simulink model "fourdrive_test"  (R2022b)
settings: Solver=FixedStepDiscrete  StartTime=0.0  StopTime=10.0  FixedStep=0.001  RelTol=1e-3  EnableMultiTasking=on
PreLoadFcn:
  | PowerOn_data
InitFcn:
  | EcoCoder_PreCheckLic();
undefined symbols (not defined in the file or in its folder): HV_Botton, Inverter_Button, SC_Closed
libraries: CoderSF_BSW_Libs x113, SF_CanService_Libs x24, CoderSF_ADC2Volt_Libs x10, simulink x2
(part 2 of 2)

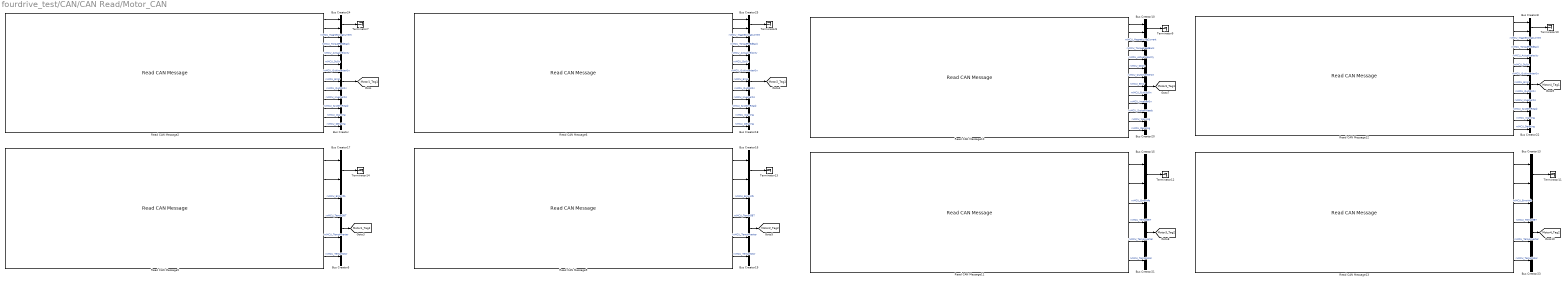
== system fourdrive_test/CAN/CAN Read/Motor_CAN ==
  Bus Creator{,18,20,22} (4 alike) : BusCreator  Inputs=11
  Bus Creator{8,10,13,15..17,24..25} (8 alike) : BusCreator  Inputs=2
  Bus Creator{5,19,21,23} (4 alike) : BusCreator  Inputs=4
  Read CAN Message10 : SF_CanService_Libs/Read CAN Message  typeCAN=Connected  channel=CAN_D  mEn=off  msgInfo=Motor_Can_All  msgItermStore=MCU_287_RL  msgIterm=MCU_287_RL  valid=on  stale=on  motoBit=off  setSignalName=on  flgCustomMonitorVariableRules=on  defineSignalName=off  prefixSignal='rx'  flgValTest=off  flgNoFixed=on  tSample=Task_Inherit  modeCode=Parameterless
  Read CAN Message11 : SF_CanService_Libs/Read CAN Message  typeCAN=Connected  channel=CAN_D  mEn=off  msgInfo=Motor_Can_All  msgItermStore=MCU_289_RL  msgIterm=MCU_289_RL  valid=on  stale=on  motoBit=off  setSignalName=on  flgCustomMonitorVariableRules=on  defineSignalName=off  prefixSignal='rx'  flgValTest=off  flgNoFixed=on  tSample=Task_Inherit  modeCode=Parameterless
  Read CAN Message12 : SF_CanService_Libs/Read CAN Message  typeCAN=Connected  channel=CAN_D  mEn=off  msgInfo=Motor_Can_All  msgItermStore=MCU_288_RR  msgIterm=MCU_288_RR  valid=on  stale=on  motoBit=off  setSignalName=on  flgCustomMonitorVariableRules=on  defineSignalName=off  prefixSignal='rx'  flgValTest=off  flgNoFixed=on  tSample=Task_Inherit  modeCode=Parameterless
  Read CAN Message13 : SF_CanService_Libs/Read CAN Message  typeCAN=Connected  channel=CAN_D  mEn=off  msgInfo=Motor_Can_All  msgItermStore=MCU_28A_RR  msgIterm=MCU_28A_RR  valid=on  stale=on  motoBit=off  setSignalName=on  flgCustomMonitorVariableRules=on  defineSignalName=off  prefixSignal='rx'  flgValTest=off  flgNoFixed=on  tSample=Task_Inherit  modeCode=Parameterless
  Read CAN Message2 : SF_CanService_Libs/Read CAN Message  typeCAN=Connected  channel=CAN_C  mEn=off  msgInfo=Motor_Can_All  msgItermStore=MCU_283_FL  msgIterm=MCU_283_FL  valid=on  stale=on  motoBit=off  setSignalName=on  flgCustomMonitorVariableRules=on  defineSignalName=off  prefixSignal='rx'  flgValTest=off  flgNoFixed=on  tSample=Task_Inherit  modeCode=Parameterless
  Read CAN Message5 : SF_CanService_Libs/Read CAN Message  typeCAN=Connected  channel=CAN_C  mEn=off  msgInfo=Motor_Can_All  msgItermStore=MCU_285_FL  msgIterm=MCU_285_FL  valid=on  stale=on  motoBit=off  setSignalName=on  flgCustomMonitorVariableRules=on  defineSignalName=off  prefixSignal='rx'  flgValTest=off  flgNoFixed=on  tSample=Task_Inherit  modeCode=Parameterless
  Read CAN Message6 : SF_CanService_Libs/Read CAN Message  typeCAN=Connected  channel=CAN_C  mEn=off  msgInfo=Motor_Can_All  msgItermStore=MCU_284_FR  msgIterm=MCU_284_FR  valid=on  stale=on  motoBit=off  setSignalName=on  flgCustomMonitorVariableRules=on  defineSignalName=off  prefixSignal='rx'  flgValTest=off  flgNoFixed=on  tSample=Task_Inherit  modeCode=Parameterless
  Read CAN Message9 : SF_CanService_Libs/Read CAN Message  typeCAN=Connected  channel=CAN_C  mEn=off  msgInfo=Motor_Can_All  msgItermStore=MCU_286_FR  msgIterm=MCU_286_FR  valid=on  stale=on  motoBit=off  setSignalName=on  flgCustomMonitorVariableRules=on  defineSignalName=off  prefixSignal='rx'  flgValTest=off  flgNoFixed=on  tSample=Task_Inherit  modeCode=Parameterless
  Terminator{7..14} (8 alike) : Terminator
  tag scope: Motor1_Tag1=global, Motor1_Tag2=global, Motor2_Tag1=global, Motor2_Tag2=global, Motor3_Tag1=global, Motor3_Tag2=global, Motor4_Tag1=global, Motor4_Tag2=global
  wires:
  Read CAN Message9/4 -> Bus Creator19/2  "rxMCU_TempIGBT"
  Read CAN Message9/1 -> Bus Creator16/1
  Bus Creator17/1 -> Terminator14/1
  Read CAN Message5/2 -> Bus Creator17/2
  Read CAN Message5/1 -> Bus Creator17/1
  Bus Creator19/1 -> [Motor2_Tag2]
  Read CAN Message11/2 -> Bus Creator15/2
  Read CAN Message12/1 -> Bus Creator8/1
  Read CAN Message2/1 -> Bus Creator24/1
  Bus Creator15/1 -> Terminator12/1
  Read CAN Message6/3 -> Bus Creator18/1  "rxMCU_MagnetizingCurrent"
  Read CAN Message12/3 -> Bus Creator22/1  "rxMCU_MagnetizingCurrent"
  Bus Creator16/1 -> Terminator13/1
  Bus Creator23/1 -> [Motor4_Tag2]
  Read CAN Message9/2 -> Bus Creator16/2
  Read CAN Message2/7 -> Bus Creator/5  "rxMCU_QuitInverterOn"
  Bus Creator/1 -> [Motor1_Tag1]
  Read CAN Message10/3 -> Bus Creator20/1  "rxMCU_MagnetizingCurrent"
  Bus Creator25/1 -> Terminator8/1
  Read CAN Message13/1 -> Bus Creator13/1
  Read CAN Message6/2 -> Bus Creator25/2
  Read CAN Message2/10 -> Bus Creator/8  "rxMCU_InverterOn"
  Bus Creator13/1 -> Terminator11/1
  Bus Creator10/1 -> Terminator9/1
  Read CAN Message6/10 -> Bus Creator18/8  "rxMCU_InverterOn"
  Read CAN Message11/1 -> Bus Creator15/1
  Read CAN Message13/3 -> Bus Creator23/1  "rxMCU_ErrorInfo"
  Read CAN Message10/2 -> Bus Creator10/2
  Read CAN Message12/2 -> Bus Creator8/2
  Bus Creator8/1 -> Terminator10/1
  Read CAN Message11/4 -> Bus Creator21/2  "rxMCU_TempIGBT"
  Read CAN Message5/3 -> Bus Creator5/1  "rxMCU_ErrorInfo"
  Read CAN Message6/12 -> Bus Creator18/10  "rxMCU_Warning"
  Read CAN Message10/7 -> Bus Creator20/5  "rxMCU_QuitInverterOn"
  Bus Creator24/1 -> Terminator7/1
  Read CAN Message2/2 -> Bus Creator24/2
  Bus Creator22/1 -> [Motor4_Tag1]
  Read CAN Message12/6 -> Bus Creator22/4  "rxMCU_DcOn"
  Read CAN Message10/11 -> Bus Creator20/9  "rxMCU_SystemReady"
  Read CAN Message2/8 -> Bus Creator/6  "rxMCU_Error"
  Read CAN Message5/4 -> Bus Creator5/2  "rxMCU_TempIGBT"
  Read CAN Message2/6 -> Bus Creator/4  "rxMCU_DcOn"
  Read CAN Message12/10 -> Bus Creator22/8  "rxMCU_InverterOn"
  Read CAN Message2/9 -> Bus Creator/7  "rxMCU_QuitDcOn"
  Read CAN Message2/3 -> Bus Creator/1  "rxMCU_MagnetizingCurrent"
  Read CAN Message6/8 -> Bus Creator18/6  "rxMCU_Error"
  Read CAN Message13/2 -> Bus Creator13/2
  Read CAN Message2/11 -> Bus Creator/9  "rxMCU_SystemReady"
  Bus Creator18/1 -> [Motor2_Tag1]
  Read CAN Message12/8 -> Bus Creator22/6  "rxMCU_Error"
  Read CAN Message6/5 -> Bus Creator18/3  "rxMCU_ActualVelocity"
  Read CAN Message12/4 -> Bus Creator22/2  "rxMCU_TorqueFeedBack"
  Read CAN Message10/13 -> Bus Creator20/11  "rxMCU_Derating"
  Read CAN Message10/12 -> Bus Creator20/10  "rxMCU_Warning"
  Read CAN Message12/13 -> Bus Creator22/11  "rxMCU_Derating"
  Read CAN Message6/7 -> Bus Creator18/5  "rxMCU_QuitInverterOn"
  Read CAN Message6/13 -> Bus Creator18/11  "rxMCU_Derating"
  Read CAN Message10/4 -> Bus Creator20/2  "rxMCU_TorqueFeedBack"
  Read CAN Message10/6 -> Bus Creator20/4  "rxMCU_DcOn"
  Read CAN Message10/10 -> Bus Creator20/8  "rxMCU_InverterOn"
  Read CAN Message10/9 -> Bus Creator20/7  "rxMCU_QuitDcOn"
  Read CAN Message12/12 -> Bus Creator22/10  "rxMCU_Warning"
  Read CAN Message12/7 -> Bus Creator22/5  "rxMCU_QuitInverterOn"
  Read CAN Message10/1 -> Bus Creator10/1
  Read CAN Message10/5 -> Bus Creator20/3  "rxMCU_ActualVelocity"
  Read CAN Message11/5 -> Bus Creator21/3  "rxMCU_TempInverter"
  Bus Creator5/1 -> [Motor1_Tag2]
  Bus Creator20/1 -> [Motor3_Tag1]
  Read CAN Message12/5 -> Bus Creator22/3  "rxMCU_ActualVelocity"
  Read CAN Message6/11 -> Bus Creator18/9  "rxMCU_SystemReady"
  Read CAN Message6/9 -> Bus Creator18/7  "rxMCU_QuitDcOn"
  Read CAN Message6/6 -> Bus Creator18/4  "rxMCU_DcOn"
  Bus Creator21/1 -> [Motor3_Tag2]
  Read CAN Message12/9 -> Bus Creator22/7  "rxMCU_QuitDcOn"
  Read CAN Message10/8 -> Bus Creator20/6  "rxMCU_Error"
  Read CAN Message13/4 -> Bus Creator23/2  "rxMCU_TempIGBT"
  Read CAN Message11/3 -> Bus Creator21/1  "rxMCU_ErrorInfo"
  Read CAN Message2/13 -> Bus Creator/11  "rxMCU_Derating"
  Read CAN Message9/3 -> Bus Creator19/1  "rxMCU_ErrorInfo"
  Read CAN Message2/12 -> Bus Creator/10  "rxMCU_Warning"
  Read CAN Message12/11 -> Bus Creator22/9  "rxMCU_SystemReady"
  Read CAN Message13/5 -> Bus Creator23/3  "rxMCU_TempInverter"
  Read CAN Message9/5 -> Bus Creator19/3  "rxMCU_TempInverter"
  Read CAN Message5/5 -> Bus Creator5/3  "rxMCU_TempInverter"
  Read CAN Message2/4 -> Bus Creator/2  "rxMCU_TorqueFeedBack"
  Read CAN Message6/4 -> Bus Creator18/2  "rxMCU_TorqueFeedBack"
  Read CAN Message2/5 -> Bus Creator/3  "rxMCU_ActualVelocity"
  Read CAN Message6/1 -> Bus Creator25/1
  Read CAN Message5/6 -> Bus Creator5/4  "rxMCU_TempMotor"
  Read CAN Message9/6 -> Bus Creator19/4  "rxMCU_TempMotor"
  Read CAN Message11/6 -> Bus Creator21/4  "rxMCU_TempMotor"
  Read CAN Message13/6 -> Bus Creator23/4  "rxMCU_TempMotor"

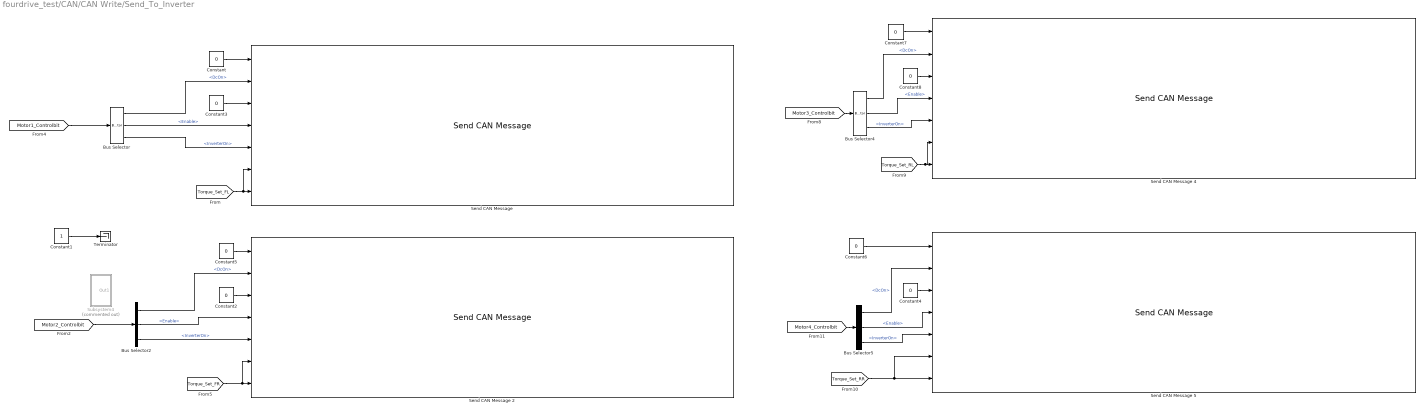
== system fourdrive_test/CAN/CAN Write/Send_To_Inverter ==
  Bus Selector{,2,4..5} (4 alike) : BusSelector  OutputSignals=DcOn,Enable,InverterOn
  Constant{,5..7} (4 alike) : Constant  Value=0  OutDataTypeStr=Inherit: Inherit via back propagation
  Constant1 : Constant
  Constant{2..4,8} (4 alike) : Constant  Value=0  OutDataTypeStr=single
  "Send CAN Message " : SF_CanService_Libs/Send CAN Message   typeCAN=Connected  channel=CAN_C  mEn=off  msgInfo=AMK_VCU_CAN_TorqueMode_factor_edited  msgItermStore=VCU1_0x184  msgIterm=VCU1_0x184  motoBit=off  flgNoFixed=on  tSample=Task_Inherit  modeCode=Parameterless  modeRound=Zero
  Send CAN Message 2 : SF_CanService_Libs/Send CAN Message   typeCAN=Connected  channel=CAN_C  mEn=off  msgInfo=AMK_VCU_CAN_TorqueMode_factor_edited  msgItermStore=VCU2_0x185  msgIterm=VCU2_0x185  motoBit=off  flgNoFixed=on  tSample=Task_Inherit  modeCode=Parameterless  modeRound=Zero
  Send CAN Message 4 : SF_CanService_Libs/Send CAN Message   typeCAN=Connected  channel=CAN_D  mEn=off  msgInfo=AMK_VCU_CAN_TorqueMode_factor_edited  msgItermStore=VCU3_0x188  msgIterm=VCU3_0x188  motoBit=off  flgNoFixed=on  tSample=Task_Inherit  modeCode=Parameterless  modeRound=Zero
  Send CAN Message 5 : SF_CanService_Libs/Send CAN Message   typeCAN=Connected  channel=CAN_D  mEn=off  msgInfo=AMK_VCU_CAN_TorqueMode_factor_edited  msgItermStore=VCU4_0x189  msgIterm=VCU4_0x189  motoBit=off  flgNoFixed=on  tSample=Task_Inherit  modeCode=Parameterless  modeRound=Zero
  Subsystem4 : Subsystem  Commented=on
  Terminator : Terminator
  wires:
  [Motor2_Controlbit] -> Bus Selector2/1
  Bus Selector4/2 -> Send CAN Message 4/4  "<Enable>"
  [Torque_Set_FL] -> "Send CAN Message "/6, "Send CAN Message "/7
  [Motor1_Controlbit] -> Bus Selector/1
  Bus Selector/1 -> "Send CAN Message "/2  "<DcOn>"
  Bus Selector4/3 -> Send CAN Message 4/5  "<InverterOn>"
  [Motor3_Controlbit] -> Bus Selector4/1
  Bus Selector2/3 -> Send CAN Message 2/5  "<InverterOn>"
  Bus Selector5/1 -> Send CAN Message 5/2  "<DcOn>"
  Bus Selector5/3 -> Send CAN Message 5/5  "<InverterOn>"
  Constant7/1 -> Send CAN Message 4/1
  [Motor4_Controlbit] -> Bus Selector5/1
  Constant5/1 -> Send CAN Message 2/1
  Bus Selector/2 -> "Send CAN Message "/4  "<Enable>"
  Bus Selector4/1 -> Send CAN Message 4/2  "<DcOn>"
  Constant/1 -> "Send CAN Message "/1
  Bus Selector5/2 -> Send CAN Message 5/4  "<Enable>"
  Bus Selector2/1 -> Send CAN Message 2/2  "<DcOn>"
  [Torque_Set_FR] -> Send CAN Message 2/6, Send CAN Message 2/7
  Bus Selector/3 -> "Send CAN Message "/5  "<InverterOn>"
  [Torque_Set_RL] -> Send CAN Message 4/6, Send CAN Message 4/7
  Bus Selector2/2 -> Send CAN Message 2/4  "<Enable>"
  [Torque_Set_RR] -> Send CAN Message 5/6, Send CAN Message 5/7
  Constant6/1 -> Send CAN Message 5/1
  Constant1/1 -> Terminator/1
  Constant3/1 -> "Send CAN Message "/3
  Constant2/1 -> Send CAN Message 2/3
  Constant4/1 -> Send CAN Message 5/3
  Constant8/1 -> Send CAN Message 4/3

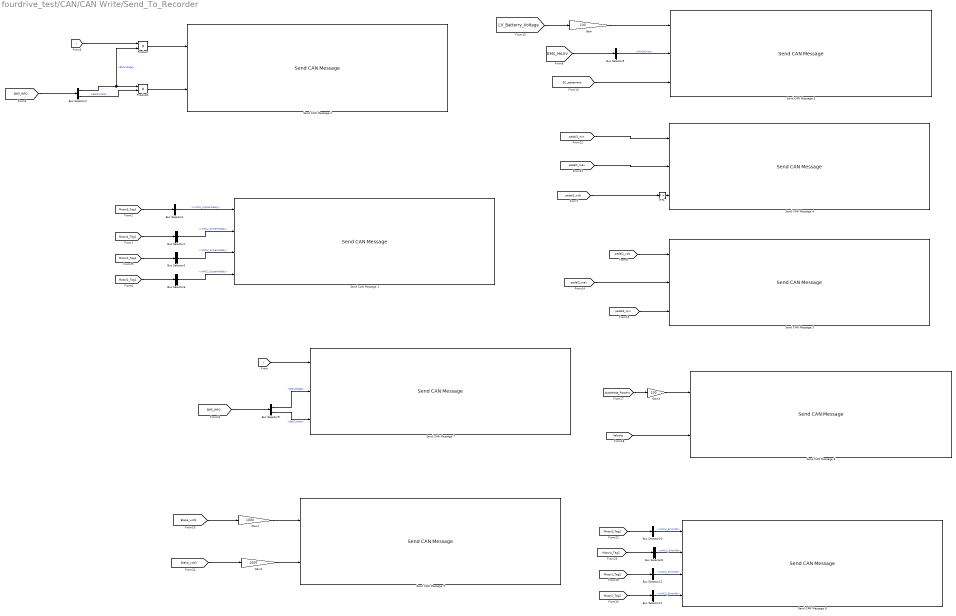
== system fourdrive_test/CAN/CAN Write/Send_To_Recorder ==
  Bus Selector{1..2,6..7} (4 alike) : BusSelector  OutputSignals=rxMCU_SystemReady
  Bus Selector{8,10..12} (4 alike) : BusSelector  OutputSignals=rxMCU_ErrorInfo
  Bus Selector3 : BusSelector  OutputSignals=BatVoltage,BatCurrent
  Bus Selector5 : BusSelector  OutputSignals=MinCellVolt
  Bus Selector9 : BusSelector  OutputSignals=BatVoltage,BatCurrent
  Gain : Gain  Gain=100  OutDataTypeStr=uint16
  Gain1 : Gain  Gain=1000  OutDataTypeStr=uint16
  Gain2 : Gain  Gain=1000  OutDataTypeStr=uint16
  Gain3 : Gain  Gain=100  ParamDataTypeStr=uint16
  Product : Product
  Product1 : Product
  RT1 : RateTransition  OutPortSampleTime=0.05
  Send CAN Message 1 : SF_CanService_Libs/Send CAN Message   typeCAN=Connected  channel=CAN_A  mEn=off  msgInfo=inventer_ready  msgItermStore=Systerm_ready  msgIterm=Systerm_ready  motoBit=off  flgNoFixed=on  tSample=Task_L100ms  modeCode=Parameterless  modeRound=Zero
  Send CAN Message 2 : SF_CanService_Libs/Send CAN Message   typeCAN=Connected  channel=CAN_A  mEn=off  msgInfo=the_different_total_power  msgItermStore=total_power  msgIterm=total_power  motoBit=off  flgNoFixed=on  tSample=Task_L100ms  modeCode=Parameterless  modeRound=Zero
  Send CAN Message 3 : SF_CanService_Libs/Send CAN Message   typeCAN=Connected  channel=CAN_A  mEn=off  msgInfo=LV_volt  msgItermStore=To_Record_SC  msgIterm=To_Record_SC  motoBit=off  flgNoFixed=on  tSample=Task_L20ms  modeCode=Parameterless  modeRound=Zero
  Send CAN Message 4 : SF_CanService_Libs/Send CAN Message   typeCAN=Connected  channel=CAN_A  mEn=off  msgInfo=pedal_and_SC  msgItermStore=To_Record_pedal1  msgIterm=To_Record_pedal1  motoBit=off  flgNoFixed=on  tSample=Task_L50ms  modeCode=Parameterless  modeRound=Zero
  Send CAN Message 5 : SF_CanService_Libs/Send CAN Message   typeCAN=Connected  channel=CAN_A  mEn=off  msgInfo=pedal_and_SC  msgItermStore=To_Recorde_pedal2  msgIterm=To_Recorde_pedal2  motoBit=off  flgNoFixed=on  tSample=Task_L50ms  modeCode=Parameterless  modeRound=Zero
  Send CAN Message 6 : SF_CanService_Libs/Send CAN Message   typeCAN=Connected  channel=CAN_A  mEn=off  msgInfo=pedal_and_SC  msgItermStore=pedal_velocity  msgIterm=pedal_velocity  motoBit=off  flgNoFixed=on  tSample=Task_L50ms  modeCode=Parameterless  modeRound=Zero
  Send CAN Message 7 : SF_CanService_Libs/Send CAN Message   typeCAN=Connected  channel=CAN_A  mEn=off  msgInfo=the_different_total_power  msgItermStore=To_Recorder_Battery  msgIterm=To_Recorder_Battery  motoBit=off  flgNoFixed=on  tSample=Task_L20ms  modeCode=Parameterless  modeRound=Zero
  Send CAN Message 8 : SF_CanService_Libs/Send CAN Message   typeCAN=Connected  channel=CAN_A  mEn=off  msgInfo=pedal_and_SC  msgItermStore=error_info  msgIterm=error_info  motoBit=off  flgNoFixed=on  tSample=Task_L100ms  modeCode=Parameterless  modeRound=Zero
  Send CAN Message 9 : SF_CanService_Libs/Send CAN Message   typeCAN=Connected  channel=CAN_A  mEn=off  msgInfo=LV_volt  msgItermStore=brake_volt  msgIterm=brake_volt  motoBit=off  flgNoFixed=on  tSample=Task_L20ms  modeCode=Parameterless  modeRound=Zero
  wires:
  [pedal1_volt] -> RT1/1
  [SC_statement] -> Send CAN Message 3/3
  [BMS_MAXV] -> Bus Selector5/1
  Bus Selector5/1 -> Send CAN Message 3/2  "<MinCellVolt>"
  [BMS_INFO] -> Bus Selector9/1
  Bus Selector9/2 -> Send CAN Message 7/3  "<BatCurrent>"
  Bus Selector9/1 -> Send CAN Message 7/2  "<BatVoltage>"
  [I] -> Send CAN Message 7/1
  [Motor1_Tag2] -> Bus Selector12/1
  [Motor2_Tag2] -> Bus Selector11/1
  [Motor3_Tag2] -> Bus Selector10/1
  [Motor4_Tag2] -> Bus Selector8/1
  Bus Selector12/1 -> Send CAN Message 8/3  "<rxMCU_ErrorInfo>"
  Bus Selector11/1 -> Send CAN Message 8/4  "<rxMCU_ErrorInfo>"
  Bus Selector10/1 -> Send CAN Message 8/1  "<rxMCU_ErrorInfo>"
  Bus Selector8/1 -> Send CAN Message 8/2  "<rxMCU_ErrorInfo>"
  [pedal1_max] -> Send CAN Message 4/2
  [pedal1_min] -> Send CAN Message 4/1
  [pedal2_max] -> Send CAN Message 5/2
  [pedal2_min] -> Send CAN Message 5/3
  [Accelerate_Percent] -> Gain3/1
  [pedal2_volt] -> Send CAN Message 5/1
  RT1/1 -> Send CAN Message 4/3
  [Velocity] -> Send CAN Message 6/2
  [LV_Batterry_Voltage] -> Gain/1
  Gain/1 -> Send CAN Message 3/1
  [Brake_volt2] -> Gain2/1
  [Brake_volt1] -> Gain1/1
  Gain1/1 -> Send CAN Message 9/1
  Gain2/1 -> Send CAN Message 9/2
  Gain3/1 -> Send CAN Message 6/1
  [Motor4_Tag1] -> Bus Selector7/1
  Bus Selector6/1 -> Send CAN Message 1/4  "<rxMCU_SystemReady>"
  Bus Selector2/1 -> Send CAN Message 1/3  "<rxMCU_SystemReady>"
  [Motor2_Tag1] -> Bus Selector6/1
  [Motor1_Tag1] -> Bus Selector2/1
  Bus Selector7/1 -> Send CAN Message 1/2  "<rxMCU_SystemReady>"
  Bus Selector1/1 -> Send CAN Message 1/1  "<rxMCU_SystemReady>"
  [Motor3_Tag1] -> Bus Selector1/1
  [I] -> Product/1
  Bus Selector3/2 -> Product1/2  "<BatCurrent>"
  [BMS_INFO] -> Bus Selector3/1
  Bus Selector3/1 -> Product/2, Product1/1  "<BatVoltage>"
  Product1/1 -> Send CAN Message 2/2
  Product/1 -> Send CAN Message 2/1

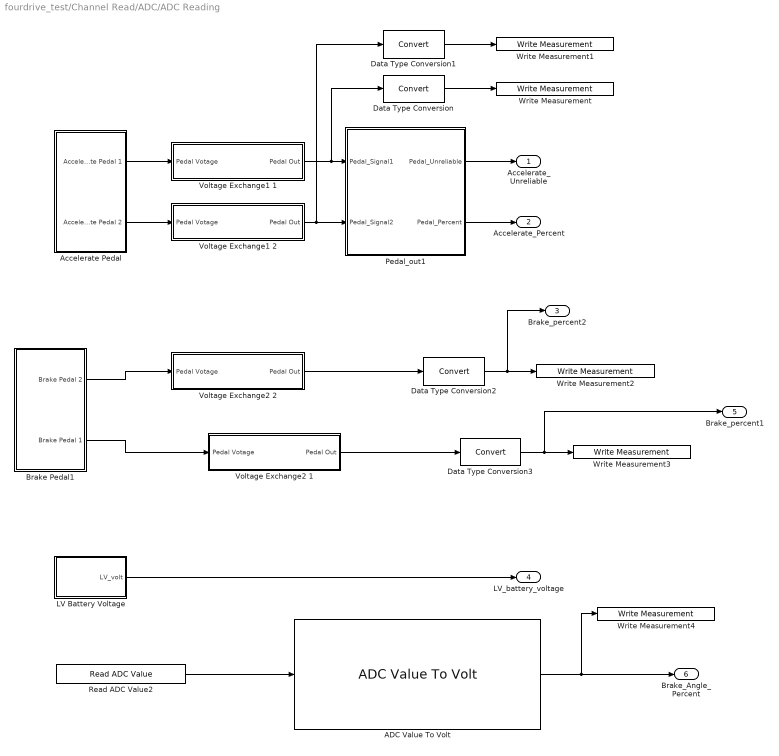
== system fourdrive_test/Channel Read/ADC/ADC Reading  ==
  ADC Value To Volt : CoderSF_ADC2Volt_Libs/ADC Value To Volt  ResValue=12  RefValue=5  TypeOut=single  WithDiv=off  DivValue=0  SerValue=22
  Accelerate Pedal : Subsystem
  Brake Pedal1 : Subsystem
  Data Type Conversion{,1..3} (4 alike) : DataTypeConversion  SaturateOnIntegerOverflow=off  RndMeth=Floor
  LV Battery Voltage : Subsystem
  Pedal_out1 : Subsystem
  Read ADC Value2 : CoderSF_BSW_Libs/ADC/Read ADC Value  channel=21
  Voltage Exchange1 1 : Subsystem
  Voltage Exchange1 2 : Subsystem
  Voltage Exchange2 1 : Subsystem
  Voltage Exchange2 2 : Subsystem
  Write Measurement : CoderSF_BSW_Libs/Calibration & Measurement/Write Measurement  variable_name=ACC_per_h  variable_value=0  variable_type=single  numD=1  unitStr=""  descStr=""
      settings: AttributesFormatString=type:%<variable_type> Dimensions:%<numD>
  Write Measurement1 : CoderSF_BSW_Libs/Calibration & Measurement/Write Measurement  variable_name=ACC_per_l  variable_value=0  variable_type=single  numD=1  unitStr=""  descStr=""
      settings: AttributesFormatString=type:%<variable_type> Dimensions:%<numD>
  Write Measurement2 : CoderSF_BSW_Libs/Calibration & Measurement/Write Measurement  variable_name=brake_per_2  variable_value=0  variable_type=single  numD=1  unitStr=""  descStr=""
      settings: AttributesFormatString=type:%<variable_type> Dimensions:%<numD>
  Write Measurement3 : CoderSF_BSW_Libs/Calibration & Measurement/Write Measurement  variable_name=brake_per_1  variable_value=0  variable_type=single  numD=1  unitStr=""  descStr=""
      settings: AttributesFormatString=type:%<variable_type> Dimensions:%<numD>
  Write Measurement4 : CoderSF_BSW_Libs/Calibration & Measurement/Write Measurement  variable_name=Brake_angle_volt  variable_value=0  variable_type=single  numD=1  unitStr=""  descStr=""
      settings: AttributesFormatString=type:%<variable_type> Dimensions:%<numD>
  Accelerate_Unreliable : Outport  VectorParamsAs1DForOutWhenUnconnected=off
  Accelerate_Percent : Outport  Port=2  VectorParamsAs1DForOutWhenUnconnected=off
  Brake_percent2 : Outport  Port=3
  LV_battery_voltage : Outport  Port=4  VectorParamsAs1DForOutWhenUnconnected=off
  Brake_percent1 : Outport  Port=5
  Brake_Angle_Percent : Outport  Port=6
  wires:
  Accelerate Pedal/1(Accelerate Pedal 1) -> Voltage Exchange1 1/1(Pedal Votage)
  Accelerate Pedal/2(Accelerate Pedal 2) -> Voltage Exchange1 2/1(Pedal Votage)
  Brake Pedal1/1(Brake Pedal 2) -> Voltage Exchange2 2/1(Pedal Votage)
  Voltage Exchange1 1/1(Pedal Out) -> Data Type Conversion/1, Pedal_out1/1(Pedal_Signal1)
  Pedal_out1/1(Pedal_Unreliable) -> Accelerate_Unreliable/1
  Pedal_out1/2(Pedal_Percent) -> Accelerate_Percent/1
  Data Type Conversion/1 -> Write Measurement/1
  Voltage Exchange1 2/1(Pedal Out) -> Data Type Conversion1/1, Pedal_out1/2(Pedal_Signal2)
  Data Type Conversion1/1 -> Write Measurement1/1
  Voltage Exchange2 2/1(Pedal Out) -> Data Type Conversion2/1
  Data Type Conversion2/1 -> Brake_percent2/1, Write Measurement2/1
  Brake Pedal1/2(Brake Pedal 1) -> Voltage Exchange2 1/1(Pedal Votage)
  Voltage Exchange2 1/1(Pedal Out) -> Data Type Conversion3/1
  Data Type Conversion3/1 -> Brake_percent1/1, Write Measurement3/1
  Read ADC Value2/1 -> ADC Value To Volt/1
  ADC Value To Volt/1 -> Write Measurement4/1, Brake_Angle_Percent/1
  LV Battery Voltage/1(LV_volt) -> LV_battery_voltage/1

== system fourdrive_test/Channel Read/ADC/DCDC_temp ==
  ADC Value To Volt : CoderSF_ADC2Volt_Libs/ADC Value To Volt  ResValue=12  RefValue=5  TypeOut=single  WithDiv=off  DivValue=0  SerValue=22
  Read ADC Value2 : CoderSF_BSW_Libs/ADC/Read ADC Value  channel=16
  Terminator : Terminator
  Write Measurement : CoderSF_BSW_Libs/Calibration & Measurement/Write Measurement  variable_name=DCDC_temp  variable_value=0  variable_type=single  numD=1  unitStr=""  descStr=""
      settings: AttributesFormatString=type:%<variable_type> Dimensions:%<numD>
  tag scope: DCDC_temp=global
  wires:
  Read ADC Value2/1 -> ADC Value To Volt/1
  ADC Value To Volt/1 -> Write Measurement/1, [DCDC_temp]
  [DCDC_temp] -> Terminator/1

== system fourdrive_test/Channel Read/ADC/安全回路模拟量 ==
  ADC Value To Volt : CoderSF_ADC2Volt_Libs/ADC Value To Volt  ResValue=12  RefValue=5  TypeOut=single  WithDiv=off  DivValue=3.48  SerValue=22
  Read ADC Value2 : CoderSF_BSW_Libs/ADC/Read ADC Value  channel=6
  Terminator : Terminator
  Write Measurement : CoderSF_BSW_Libs/Calibration & Measurement/Write Measurement  variable_name=SC_statement  variable_value=0  variable_type=single  numD=1  unitStr=""  descStr=""
      settings: AttributesFormatString=type:%<variable_type> Dimensions:%<numD>
  tag scope: SC_statement=global
  wires:
  ADC Value To Volt/1 -> Write Measurement/1
  Read ADC Value2/1 -> [SC_statement], ADC Value To Volt/1
  [SC_statement] -> Terminator/1

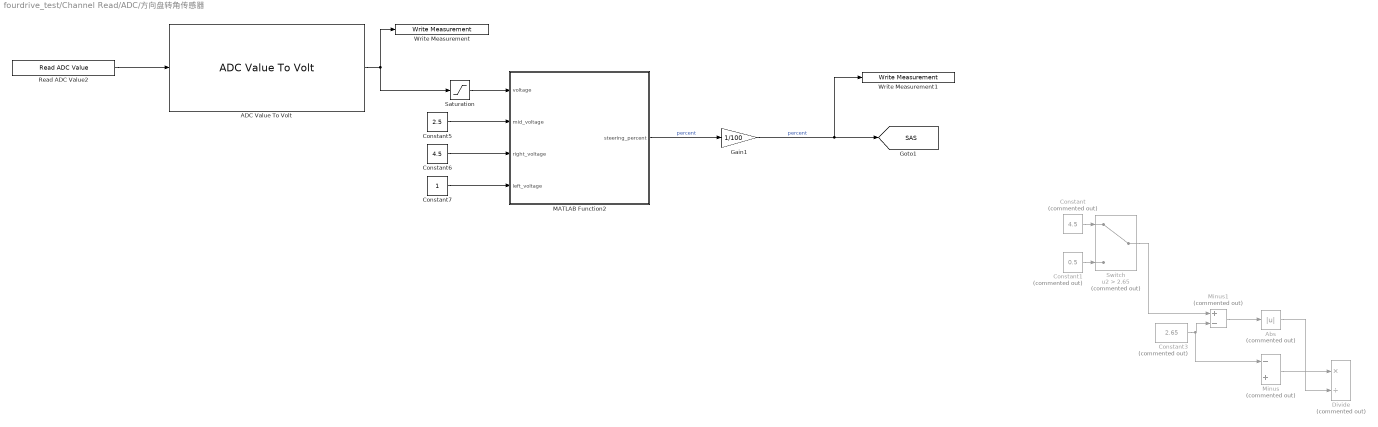
== system fourdrive_test/Channel Read/ADC/方向盘转角传感器 ==
  ADC Value To Volt : CoderSF_ADC2Volt_Libs/ADC Value To Volt  ResValue=12  RefValue=5  TypeOut=single  WithDiv=off  DivValue=0  SerValue=22
  Abs : Abs  Commented=on  SaturateOnIntegerOverflow=off
  Constant : Constant  Commented=on  Value=4.5
  Constant1 : Constant  Commented=on  Value=0.5
  Constant3 : Constant  Commented=on  Value=2.65
  Constant5 : Constant  Value=2.5
  Constant6 : Constant  Value=4.5
  Constant7 : Constant
  Divide : Product  Commented=on  Inputs=*/  OutDataTypeStr=single
  Gain1 : Gain  Gain=1/100  OutDataTypeStr=single
  MATLAB Function2 : MATLAB Function  TreatAsAtomicUnit=on
  Minus : Sum  Commented=on  Inputs=-+
  Minus1 : Sum  Commented=on  Inputs=+-
  Read ADC Value2 : CoderSF_BSW_Libs/ADC/Read ADC Value  channel=15
  Saturation : Saturate  UpperLimit=5  LowerLimit=0
  Switch : Switch  Commented=on  Criteria=u2 > Threshold  Threshold=2.65  SaturateOnIntegerOverflow=off  InputSameDT=off
  Write Measurement : CoderSF_BSW_Libs/Calibration & Measurement/Write Measurement  variable_name=steering_volt  variable_value=0  variable_type=single  numD=1  unitStr=""  descStr=""
      settings: AttributesFormatString=type:%<variable_type> Dimensions:%<numD>
  Write Measurement1 : CoderSF_BSW_Libs/Calibration & Measurement/Write Measurement  variable_name=steering_angle  variable_value=0  variable_type=single  numD=1  unitStr=""  descStr=""
      settings: AttributesFormatString=type:%<variable_type> Dimensions:%<numD>
  tag scope: SAS=global
  wires:
  Read ADC Value2/1 -> ADC Value To Volt/1
  ADC Value To Volt/1 -> Saturation/1, Write Measurement/1
  Constant/1 -> Switch/1
  Constant3/1 -> Minus/1, Minus1/2
  Minus/1 -> Divide/1
  Abs/1 -> Divide/2
  Switch/1 -> Minus1/1
  Constant1/1 -> Switch/3
  Minus1/1 -> Abs/1
  Constant5/1 -> MATLAB Function2/2(mid_voltage)
  MATLAB Function2/1(steering_percent) -> Gain1/1  "percent"
  Constant7/1 -> MATLAB Function2/4(left_voltage)
  Constant6/1 -> MATLAB Function2/3(right_voltage)
  Saturation/1 -> MATLAB Function2/1(voltage)
  Gain1/1 -> Write Measurement1/1, [SAS]  "percent"

== system fourdrive_test/Channel Read/ADC/电流传感器 ==
  ADC Value To Volt : CoderSF_ADC2Volt_Libs/ADC Value To Volt  ResValue=12  RefValue=5  TypeOut=single  WithDiv=off  DivValue=0  SerValue=22
  Read ADC Value2 : CoderSF_BSW_Libs/ADC/Read ADC Value  channel=4
  Terminator : Terminator
  Write Measurement : CoderSF_BSW_Libs/Calibration & Measurement/Write Measurement  variable_name=I  variable_value=0  variable_type=single  numD=1  unitStr=""  descStr=""
      settings: AttributesFormatString=type:%<variable_type> Dimensions:%<numD>
  tag scope: I=global
  wires:
  Read ADC Value2/1 -> ADC Value To Volt/1
  ADC Value To Volt/1 -> Write Measurement/1, [I]
  [I] -> Terminator/1

== system fourdrive_test/Control/Torque_Control/Subsystem ==
  In1 : Inport
  Constant4 : Constant  Value=0  OutDataTypeStr=uint16
  Switch3 : Switch  Criteria=u2 > Threshold  SaturateOnIntegerOverflow=off  InputSameDT=off
  Out1 : Outport
  wires:
  [ready_F] -> Switch3/2
  Constant4/1 -> Switch3/3
  Switch3/1 -> Out1/1
  In1/1 -> Switch3/1

== system fourdrive_test/Control/Torque_Control/Subsystem1 ==
  In1 : Inport
  Constant4 : Constant  Value=0  OutDataTypeStr=uint16
  Switch3 : Switch  Criteria=u2 > Threshold  SaturateOnIntegerOverflow=off  InputSameDT=off
  Out1 : Outport
  wires:
  [ready_F] -> Switch3/2
  Constant4/1 -> Switch3/3
  Switch3/1 -> Out1/1
  In1/1 -> Switch3/1

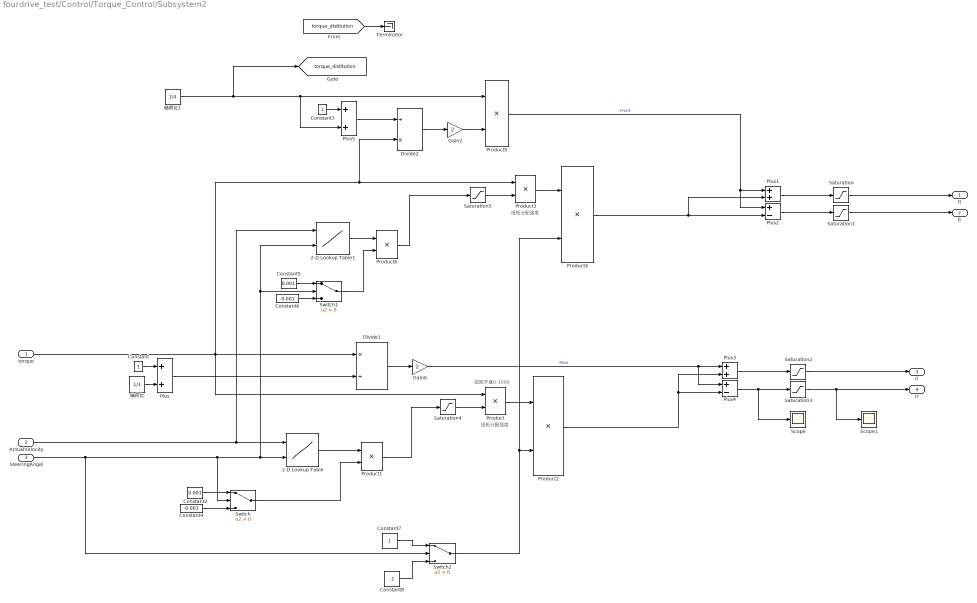
== system fourdrive_test/Control/Torque_Control/Subsystem2 ==
  note: 扭矩分配强度
  note: 扭矩开度0-1000
  note: 扭矩分配强度
  torque : Inport
  ActualVelocity : Inport  Port=2
  SteeringAngel : Inport  Port=3
  2-D Lookup Table : Lookup_n-D  BreakpointsSpecification=Even spacing  BreakpointsForDimension1=[-180:180]  BreakpointsForDimension2=[2000:18000]  BreakpointsForDimension1FirstPoint=0  BreakpointsForDimension2FirstPoint=0  BreakpointsForDimension1Spacing=3000  BreakpointsForDimension2Spacing=30  BreakpointsForDimension1DataTypeStr=single  BreakpointsForDimension2DataTypeStr=double  Table=[0 60 90 150 240 270 300;0 60 90 150 240 270 300;0 60 90 150 240 270 300;0 60 90 150 240 270 300;0 60 90 150 240 270 300;0 0 0 0 0 0 0;0 0 0 0 0 0 0;0 0 0 0 0 0 0]  TableDataTypeStr=Inherit: Inherit from 'Table data'  ExtrapMethod=Clip  UseLastTableValue=on  InternalRulePriority=Speed  OutDataTypeStr=double  RndMeth=Simplest
      settings: InputPortMap=u0,u1
  2-D Lookup Table1 : Lookup_n-D  BreakpointsSpecification=Even spacing  BreakpointsForDimension1=[-180:180]  BreakpointsForDimension2=[2000:18000]  BreakpointsForDimension1FirstPoint=0  BreakpointsForDimension2FirstPoint=0  BreakpointsForDimension1Spacing=3000  BreakpointsForDimension2Spacing=30  BreakpointsForDimension1DataTypeStr=single  BreakpointsForDimension2DataTypeStr=single  Table=[0 72 108 180 288 324 360;0 72 108 180 288 324 360;0 72 108 180 288 324 360;0 72 108 180 288 324 360;0 72 108 180 288 324 360;0 0 0 0 0 0 0;0 0 0 0 0 0 0;0 0 0 0 0 0 0]  ExtrapMethod=Clip  UseLastTableValue=on  InternalRulePriority=Speed  OutDataTypeStr=double  RndMeth=Simplest
      settings: InputPortMap=u0,u1
  Constant : Constant
  Constant2 : Constant  Value=0.001
  Constant3 : Constant
  Constant4 : Constant  Value=-0.001
  Constant5 : Constant  Value=0.001
  Constant6 : Constant  Value=-0.001
  Constant7 : Constant
  Constant8 : Constant  Value=-1
  Divide1 : Product  Inputs=*/
  Divide2 : Product  Inputs=/*
  Gain2 : Gain  Gain=2
  Gain6 : Gain  Gain=2
  Plus{,1,3,5} (4 alike) : Sum
  Plus2 : Sum  Inputs=+-
  Plus4 : Sum  Inputs=+-
  Product{,1..6} (7 alike) : Product
  Saturation{,1..3} (4 alike) : Saturate  UpperLimit=1800  LowerLimit=0  OutDataTypeStr=uint16
  Saturation4 : Saturate  UpperLimit=0.3  LowerLimit=-0.3  OutDataTypeStr=single
  Saturation5 : Saturate  UpperLimit=0.3  LowerLimit=-0.3  OutDataTypeStr=single
  Scope : Scope
  Scope1 : Scope
  Switch : Switch  Criteria=u2 > Threshold  SaturateOnIntegerOverflow=off  InputSameDT=off
  Switch1 : Switch  Criteria=u2 > Threshold  SaturateOnIntegerOverflow=off  InputSameDT=off
  Switch2 : Switch  Criteria=u2 > Threshold  SaturateOnIntegerOverflow=off  InputSameDT=off
  Terminator : Terminator
  轴荷比 : Constant  Value=1/1
  轴荷比1 : Constant  Value=1/4
  fl : Outport
  fr : Outport  Port=2
  rl : Outport  Port=3
  rr : Outport  Port=4
  tag scope: torque_distitution=global
  wires:
  Product/1 -> Product2/1
  Saturation3/1 -> Scope1/1, rr/1
  Saturation2/1 -> rl/1
  Saturation1/1 -> fr/1
  Plus/1 -> Divide1/2
  Divide1/1 -> Gain6/1
  Plus4/1 -> Scope/1, Saturation3/1
  Plus2/1 -> Saturation1/1
  Plus1/1 -> Saturation/1
  Plus3/1 -> Saturation2/1
  Product2/1 -> Plus4/2, Plus3/2
  Gain6/1 -> Plus3/1, Plus4/1  "Rear"
  Product5/1 -> Plus1/1, Plus2/1  "Front"
  Constant/1 -> Plus/1
  Saturation/1 -> fl/1
  轴荷比/1 -> Plus/2
  Saturation4/1 -> Product/2
  Product6/1 -> Saturation5/1
  2-D Lookup Table1/1 -> Product6/1
  ActualVelocity/1 -> 2-D Lookup Table1/1, 2-D Lookup Table/1
  Product3/1 -> Product4/1
  Switch2/1 -> Product4/2, Product2/2
  Saturation5/1 -> Product3/2
  Product4/1 -> Plus1/2, Plus2/2
  Divide2/1 -> Gain2/1
  轴荷比1/1 -> [torque_distitution], Product5/1, Plus5/2
  Gain2/1 -> Product5/2
  torque/1 -> Product3/1, Divide2/2, Product/1, Divide1/1
  Constant3/1 -> Plus5/1
  Plus5/1 -> Divide2/1
  Constant2/1 -> Switch/1
  Constant4/1 -> Switch/3
  Switch/1 -> Product1/2
  2-D Lookup Table/1 -> Product1/1
  Product1/1 -> Saturation4/1
  Constant5/1 -> Switch1/1
  Constant6/1 -> Switch1/3
  Switch1/1 -> Product6/2
  Constant8/1 -> Switch2/3
  SteeringAngel/1 -> Switch2/2, Switch/2, Switch1/2, 2-D Lookup Table1/2, 2-D Lookup Table/2
  Constant7/1 -> Switch2/1
  [torque_distitution] -> Terminator/1

== system fourdrive_test/Control/Torque_Control/Subsystem4 ==
  In1 : Inport
  Constant4 : Constant  Value=0  OutDataTypeStr=uint16
  Switch3 : Switch  Criteria=u2 > Threshold  SaturateOnIntegerOverflow=off  InputSameDT=off
  Out1 : Outport
  wires:
  [ready_R] -> Switch3/2
  Constant4/1 -> Switch3/3
  Switch3/1 -> Out1/1
  In1/1 -> Switch3/1

== system fourdrive_test/Control/Torque_Control/Subsystem5 ==
  In1 : Inport
  Constant4 : Constant  Value=0  OutDataTypeStr=uint16
  Switch3 : Switch  Criteria=u2 > Threshold  SaturateOnIntegerOverflow=off  InputSameDT=off
  Out1 : Outport
  wires:
  [ready_R] -> Switch3/2
  Constant4/1 -> Switch3/3
  Switch3/1 -> Out1/1
  In1/1 -> Switch3/1

== system fourdrive_test/CAN/CAN Write/Send_To_Inverter/Subsystem4 ==
  Constant2 : Constant  OutDataTypeStr=single
  Constant3 : Constant  Value=0  OutDataTypeStr=single
  Switch : Switch  Criteria=u2 > Threshold  SaturateOnIntegerOverflow=off  InputSameDT=off
  Out1 : Outport
  wires:
  Constant3/1 -> Switch/1
  [ready_fl] -> Switch/2
  Constant2/1 -> Switch/3
  Switch/1 -> Out1/1

== system fourdrive_test/Channel Read/ADC/ADC Reading /Accelerate Pedal ==
  ADC Value To Volt : CoderSF_ADC2Volt_Libs/ADC Value To Volt  ResValue=12  RefValue=5  TypeOut=single  WithDiv=off  DivValue=0  SerValue=22
  ADC Value To Volt1 : CoderSF_ADC2Volt_Libs/ADC Value To Volt  ResValue=12  RefValue=5  TypeOut=single  WithDiv=off  DivValue=0  SerValue=22
  Read ADC Value : CoderSF_BSW_Libs/ADC/Read ADC Value  channel=1
  Read ADC Value1 : CoderSF_BSW_Libs/ADC/Read ADC Value  channel=20
  Write Measurement : CoderSF_BSW_Libs/Calibration & Measurement/Write Measurement  variable_name=ACC_Pedal_ADC1  variable_value=0  variable_type=single  numD=1  unitStr=""  descStr=""
      settings: AttributesFormatString=type:%<variable_type> Dimensions:%<numD>
  Write Measurement1 : CoderSF_BSW_Libs/Calibration & Measurement/Write Measurement  variable_name=ACC_Pedal_ADC2  variable_value=0  variable_type=single  numD=1  unitStr=""  descStr=""
      settings: AttributesFormatString=type:%<variable_type> Dimensions:%<numD>
  Accelerate Pedal 1 : Outport  VectorParamsAs1DForOutWhenUnconnected=off
  Accelerate Pedal 2 : Outport  Port=2  VectorParamsAs1DForOutWhenUnconnected=off
  tag scope: pedal1_volt=global, pedal2_volt=global
  wires:
  ADC Value To Volt1/1 -> Write Measurement1/1, Accelerate Pedal 2/1
  ADC Value To Volt/1 -> Write Measurement/1, Accelerate Pedal 1/1
  Read ADC Value1/1 -> [pedal2_volt], ADC Value To Volt1/1
  Read ADC Value/1 -> [pedal1_volt], ADC Value To Volt/1

== system fourdrive_test/Channel Read/ADC/ADC Reading /Brake Pedal1 ==
  ADC Value To Volt1 : CoderSF_ADC2Volt_Libs/ADC Value To Volt  ResValue=12  RefValue=5  TypeOut=single  WithDiv=off  DivValue=0  SerValue=22
  ADC Value To Volt2 : CoderSF_ADC2Volt_Libs/ADC Value To Volt  ResValue=12  RefValue=5  TypeOut=single  WithDiv=off  DivValue=0  SerValue=22
  Data Type Conversion1 : DataTypeConversion  SaturateOnIntegerOverflow=off  RndMeth=Floor
  Data Type Conversion2 : DataTypeConversion  SaturateOnIntegerOverflow=off  RndMeth=Floor
  Read ADC Value1 : CoderSF_BSW_Libs/ADC/Read ADC Value  channel=3
  Read ADC Value2 : CoderSF_BSW_Libs/ADC/Read ADC Value  channel=5
  Write Measurement1 : CoderSF_BSW_Libs/Calibration & Measurement/Write Measurement  variable_name=brake_voltage__1  variable_value=0  variable_type=single  numD=1  unitStr=""  descStr=""
      settings: AttributesFormatString=type:%<variable_type> Dimensions:%<numD>
  Write Measurement2 : CoderSF_BSW_Libs/Calibration & Measurement/Write Measurement  variable_name=brake_voltage__2  variable_value=0  variable_type=single  numD=1  unitStr=""  descStr=""
      settings: AttributesFormatString=type:%<variable_type> Dimensions:%<numD>
  Brake Pedal 2 : Outport  VectorParamsAs1DForOutWhenUnconnected=off
  Brake Pedal 1 : Outport  Port=2  VectorParamsAs1DForOutWhenUnconnected=off
  tag scope: Brake_volt1=global, Brake_volt2=global
  wires:
  Read ADC Value1/1 -> ADC Value To Volt1/1
  ADC Value To Volt1/1 -> [Brake_volt2], Data Type Conversion2/1, Brake Pedal 2/1
  Data Type Conversion2/1 -> Write Measurement2/1
  ADC Value To Volt2/1 -> [Brake_volt1], Data Type Conversion1/1, Brake Pedal 1/1
  Data Type Conversion1/1 -> Write Measurement1/1
  Read ADC Value2/1 -> ADC Value To Volt2/1

== system fourdrive_test/Channel Read/ADC/ADC Reading /LV Battery Voltage ==
  ADC Value To Volt : CoderSF_ADC2Volt_Libs/ADC Value To Volt  ResValue=12  RefValue=32  TypeOut=single  WithDiv=on  DivValue=22  SerValue=3.48
  Read ADC Value2 : CoderSF_BSW_Libs/ADC/Read ADC Value  channel=28
  Write Measurement : CoderSF_BSW_Libs/Calibration & Measurement/Write Measurement  variable_name=LV_volt  variable_value=0  variable_type=single  numD=1  unitStr=""  descStr=""
      settings: AttributesFormatString=type:%<variable_type> Dimensions:%<numD>
  LV_volt : Outport
  wires:
  Read ADC Value2/1 -> ADC Value To Volt/1
  ADC Value To Volt/1 -> Write Measurement/1, LV_volt/1

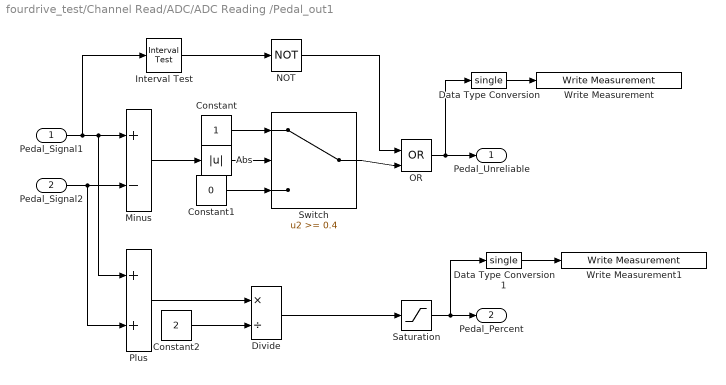
== system fourdrive_test/Channel Read/ADC/ADC Reading /Pedal_out1 ==
  Pedal_Signal1 : Inport
  Pedal_Signal2 : Inport  Port=2
  Abs : Abs  SaturateOnIntegerOverflow=off
  Constant : Constant  OutDataTypeStr=boolean
  Constant1 : Constant  Value=0  OutDataTypeStr=boolean
  Constant2 : Constant  Value=2
  Data Type Conversion : DataTypeConversion  OutDataTypeStr=single  SaturateOnIntegerOverflow=off  RndMeth=Floor
  Data Type Conversion1 : DataTypeConversion  OutDataTypeStr=single  SaturateOnIntegerOverflow=off  RndMeth=Floor
  Divide : Product  Inputs=*/
  Interval Test : simulink/Logic and Bit Operations/Interval Test  IntervalClosedRight=on  uplimit=1.2  IntervalClosedLeft=on  lowlimit=-0.2  OutDataTypeStr=boolean
  Minus : Sum  Inputs=+-
  NOT : Logic  Operator=NOT  IconShape=distinctive  AllPortsSameDT=off  OutDataTypeStr=boolean
  OR : Logic  Operator=OR  IconShape=distinctive  AllPortsSameDT=off  OutDataTypeStr=boolean
  Plus : Sum
  Saturation : Saturate  UpperLimit=1  LowerLimit=0  OutDataTypeStr=double
  Switch : Switch  Threshold=0.4  OutDataTypeStr=boolean  SaturateOnIntegerOverflow=off  InputSameDT=off
  Write Measurement : CoderSF_BSW_Libs/Calibration & Measurement/Write Measurement  variable_name=Pedal_Unreliable  variable_value=0  variable_type=single  numD=1  unitStr=""  descStr=""
      settings: AttributesFormatString=type:%<variable_type> Dimensions:%<numD>
  Write Measurement1 : CoderSF_BSW_Libs/Calibration & Measurement/Write Measurement  variable_name=Pedal_percent  variable_value=0  variable_type=single  numD=1  unitStr=""  descStr=""
      settings: AttributesFormatString=type:%<variable_type> Dimensions:%<numD>
  Pedal_Unreliable : Outport  VectorParamsAs1DForOutWhenUnconnected=off
  Pedal_Percent : Outport  Port=2  VectorParamsAs1DForOutWhenUnconnected=off
  wires:
  Pedal_Signal1/1 -> Interval Test/1, Plus/1, Minus/1
  Pedal_Signal2/1 -> Plus/2, Minus/2
  Abs/1 -> Switch/2
  Constant/1 -> Switch/1
  Constant1/1 -> Switch/3
  Plus/1 -> Divide/1
  Constant2/1 -> Divide/2
  Switch/1 -> OR/2
  OR/1 -> Data Type Conversion/1, Pedal_Unreliable/1
  Interval Test/1 -> NOT/1
  Divide/1 -> Saturation/1
  Saturation/1 -> Data Type Conversion1/1, Pedal_Percent/1
  NOT/1 -> OR/1
  Minus/1 -> Abs/1
  Data Type Conversion/1 -> Write Measurement/1
  Data Type Conversion1/1 -> Write Measurement1/1

== system fourdrive_test/Channel Read/ADC/ADC Reading /Voltage Exchange1 1 ==
  Pedal Votage : Inport
  Constant2 : Constant  Value=2.05
  Constant3 : Constant  Value=2.44
  Divide : Product  Inputs=*/
  Gain : Gain  Gain=100
  Gain1 : Gain  Gain=100
  Minus : Sum  Inputs=-+
  Minus1 : Sum  Inputs=+-
  Pedal Out : Outport  VectorParamsAs1DForOutWhenUnconnected=off
  tag scope: pedal1_max=global, pedal1_min=global
  wires:
  Minus/1 -> Divide/1
  Divide/1 -> Pedal Out/1
  Pedal Votage/1 -> Minus/2
  Constant2/1 -> Gain/1, Minus1/1
  Constant3/1 -> Gain1/1, Minus/1, Minus1/2
  Minus1/1 -> Divide/2
  Gain/1 -> [pedal1_max]
  Gain1/1 -> [pedal1_min]

== system fourdrive_test/Channel Read/ADC/ADC Reading /Voltage Exchange1 2 ==
  Pedal Votage : Inport
  Constant2 : Constant  Value=1.35
  Constant3 : Constant  Value=0.98
  Divide : Product  Inputs=*/
  Gain : Gain  Gain=100
  Gain1 : Gain  Gain=100
  Minus : Sum  Inputs=+-
  Minus1 : Sum  Inputs=+-
  Pedal Out : Outport  VectorParamsAs1DForOutWhenUnconnected=off
  tag scope: pedal2_max=global, pedal2_min=global
  wires:
  Minus/1 -> Divide/1
  Pedal Votage/1 -> Minus/1
  Divide/1 -> Pedal Out/1
  Minus1/1 -> Divide/2
  Constant3/1 -> Gain/1, Minus1/2, Minus/2
  Constant2/1 -> Gain1/1, Minus1/1
  Gain/1 -> [pedal2_min]
  Gain1/1 -> [pedal2_max]

== system fourdrive_test/Channel Read/ADC/ADC Reading /Voltage Exchange2 1 ==
  Pedal Votage : Inport
  Constant : Constant  Value=0.488
  Constant1 : Constant  Value=0.5
  Divide : Product  Inputs=*/
  Minus : Sum  Inputs=+-
  Pedal Out : Outport  VectorParamsAs1DForOutWhenUnconnected=off
  wires:
  Constant1/1 -> Divide/2
  Constant/1 -> Minus/2
  Minus/1 -> Divide/1
  Pedal Votage/1 -> Minus/1
  Divide/1 -> Pedal Out/1

== system fourdrive_test/Channel Read/ADC/ADC Reading /Voltage Exchange2 2 ==
  Pedal Votage : Inport
  Constant : Constant  Value=0.488
  Constant1 : Constant  Value=0.5
  Divide : Product  Inputs=*/
  Minus : Sum  Inputs=+-
  Pedal Out : Outport  VectorParamsAs1DForOutWhenUnconnected=off
  wires:
  Constant1/1 -> Divide/2
  Constant/1 -> Minus/2
  Minus/1 -> Divide/1
  Pedal Votage/1 -> Minus/1
  Divide/1 -> Pedal Out/1

== matlab function fourdrive_test/Channnel Out/蜂鸣器/MATLAB Function ==
  data: invertor input; count output
function count = counter_with_reset(invertor)
    % 定义持久变量存储计数状态
    persistent current_count;
    
    % 初始化计数变量
    if isempty(current_count)
        current_count = 0;
    end
    
    % 当invertor为1时递增计数，为0时重置为0
    if invertor == 1
        current_count = current_count + 1;
    else
        current_count = 0;  % invertor为0时重置计数
    end
    
    % 输出当前计数值
    count = current_count;
end

== stateflow chart fourdrive_test/Channnel Out/DC板/Chart ==
  state disabled
    DCDC_enable=false;
  state enabled
    DCDC_enable=true;
  (default) -> disabled
  disabled -> enabled : [Vehicle_Status==2&&LV_volt<26]
  enabled -> disabled : [Vehicle_Status==0]
  data: Vehicle_Status input single; DCDC_enable output boolean; LV_volt input single

== matlab function fourdrive_test/Channel Read/ADC/方向盘转角传感器/MATLAB Function2 ==
  data: voltage input; steering_percent output; mid_voltage input; right_voltage input; left_voltage input
function steering_percent = calculate_steering(voltage, mid_voltage, right_voltage, left_voltage)
% 计算转向百分比（输出限定为single类型）
% 输入:
%   voltage: 转角传感器电压(0-5V)
%   mid_voltage: 中间位置电压(例如2.65)
%   right_voltage: 右侧极限位置电压
%   left_voltage: 左侧极限位置电压
% 输出:
%   steering_percent: 转向百分比(右侧为正，范围[-100, 100]，single类型)

    % 死区范围设置(2.55-2.75V对应中间电压2.65V)
    deadband_low = mid_voltage - 0.4;
    deadband_high = mid_voltage + 0.4;
    
    % 电压钳位到0-5V范围，并转换为single类型处理
    voltage_clamped = single(max(0, min(5, voltage)));
    
    % 初始化输出为single类型的0
    steering_percent = single(0);
    
    if voltage_clamped > deadband_high
        % 右侧转向计算（向右为正）
        excess_voltage = voltage_clamped - single(deadband_high);
        max_right_voltage = single(right_voltage) - single(deadband_high);
        % 防止除以0（极限情况处理）
        if max_right_voltage <= 0
            steering_percent = single(100);
        else
            steering_percent = min(single(100), (excess_voltage / max_right_voltage) * single(100));
        end
    elseif voltage_clamped < deadband_low
        % 左侧转向计算（向左为负）
        excess_voltage = single(deadband_low) - voltage_clamped;
        max_left_voltage = single(deadband_low) - single(left_voltage);
        % 防止除以0（极限情况处理）
        if max_left_voltage <= 0
            steering_percent = single(-100);
        else
            steering_percent = max(single(-100), -(excess_voltage / max_left_voltage) * single(100));
        end
    end
    % 死区内保持初始值0（single类型）
end

== matlab function fourdrive_test/Control/Motor_Enable/MATLAB Function1 ==
  data: bSystemReady input; DcOn output; bDcOn input; bQuitDcOn input; bInverterOn input; bQuitInverterOn input; Inverter_Enable input; Enable output int16; InverterOn output int16; Ready output int16
function [DcOn, Enable, InverterOn, Ready]= Invertor( bSystemReady, bDcOn, bQuitDcOn, bInverterOn, bQuitInverterOn, Inverter_Enable)
DcOn       = int16(0);
Enable     = int16(0);
InverterOn = int16(0);
Ready      = int16(0);
if(Inverter_Enable == 1)
    if(bSystemReady    == 1)
        DcOn = int16(1);
        if(bDcOn == 1&&bQuitDcOn == 1)
            Enable     = int16(1);
            InverterOn = int16(1);
            if(bInverterOn == 1&&bQuitInverterOn == 1)
                Ready = int16(1);
            end
        end
    end
else
    DcOn = int16(1);
    Enable     = int16(0);
    InverterOn = int16(0);
    Ready = int16(0);
    if(bInverterOn == 1||bQuitInverterOn == 0)
        DcOn = int16(0);
    end
end

== matlab function fourdrive_test/Control/Motor_Enable/MATLAB Function ==
  data: bSystemReady input; DcOn output; bDcOn input; bQuitDcOn input; bInverterOn input; bQuitInverterOn input; Inverter_Enable input; Enable output int16; InverterOn output int16; Ready output int16
function [DcOn, Enable, InverterOn, Ready]= Invertor( bSystemReady, bDcOn, bQuitDcOn, bInverterOn, bQuitInverterOn, Inverter_Enable)
DcOn       = int16(0);
Enable     = int16(0);
InverterOn = int16(0);
Ready      = int16(0);
if(Inverter_Enable == 1)
    if(bSystemReady    == 1)
        DcOn = int16(1);
        if(bDcOn == 1&&bQuitDcOn == 1)
            Enable     = int16(1);
            InverterOn = int16(1);
            if(bInverterOn == 1&&bQuitInverterOn == 1)
                Ready = int16(1);
            end
        end
    end
else
    DcOn = int16(1);
    Enable     = int16(0);
    InverterOn = int16(0);
    Ready = int16(0);
    if(bInverterOn == 1||bQuitInverterOn == 0)
        DcOn = int16(0);
    end
end

== stateflow chart fourdrive_test/Control/StateMachine/Chart ==
  state LV
    Vehicle_Status=0;
  state HV
    Vehicle_Status=1;
  state DRIVE
    Vehicle_Status=2;
  (default) -> LV
  HV -> DRIVE [order 2] : [Invertor_Button==1&&SC_Closed==1 && Pedal_Unrelible==0&&Brake_enable==1 ]{Invertor_Enable=1;}
  LV -> HV : [HV_Button==1&&SC_Closed==1 && Pedal_Unrelible==0]{HV_Enable=1;}
  HV -> LV [order 1] : [SC_Closed==0]{HV_Enable=0;}
  DRIVE -> HV : [SC_Closed==0]{Invertor_Enable=0;}
  data: Vehicle_Status output; HV_Enable output; Invertor_Enable output; HV_Button input; Invertor_Button input; SC_Closed input; Pedal_Unrelible input; Brake_enable input; Accelerate_Percent input

== matlab function fourdrive_test/Control/Motor_Enable/MATLAB Function2 ==
  data: bSystemReady input; DcOn output; bDcOn input; bQuitDcOn input; bInverterOn input; bQuitInverterOn input; Inverter_Enable input; Enable output int16; InverterOn output int16; Ready output int16
function [DcOn, Enable, InverterOn, Ready]= Invertor( bSystemReady, bDcOn, bQuitDcOn, bInverterOn, bQuitInverterOn, Inverter_Enable)
DcOn       = int16(0);
Enable     = int16(0);
InverterOn = int16(0);
Ready      = int16(0);
if(Inverter_Enable == 1)
    if(bSystemReady    == 1)
        DcOn = int16(1);
        if(bDcOn == 1&&bQuitDcOn == 1)
            Enable     = int16(1);
            InverterOn = int16(1);
            if(bInverterOn == 1&&bQuitInverterOn == 1)
                Ready = int16(1);
            end
        end
    end
else
    DcOn = int16(1);
    Enable     = int16(0);
    InverterOn = int16(0);
    Ready = int16(0);
    if(bInverterOn == 1||bQuitInverterOn == 0)
        DcOn = int16(0);
    end
end

== matlab function fourdrive_test/Control/Motor_Enable/MATLAB Function3 ==
  data: bSystemReady input; DcOn output; bDcOn input; bQuitDcOn input; bInverterOn input; bQuitInverterOn input; Inverter_Enable input; Enable output int16; InverterOn output int16; Ready output int16
function [DcOn, Enable, InverterOn, Ready]= Invertor( bSystemReady, bDcOn, bQuitDcOn, bInverterOn, bQuitInverterOn, Inverter_Enable)
DcOn       = int16(0);
Enable     = int16(0);
InverterOn = int16(0);
Ready      = int16(0);
if(Inverter_Enable == 1)
    if(bSystemReady    == 1)
        DcOn = int16(1);
        if(bDcOn == 1&&bQuitDcOn == 1)
            Enable     = int16(1);
            InverterOn = int16(1);
            if(bInverterOn == 1&&bQuitInverterOn == 1)
                Ready = int16(1);
            end
        end
    end
else
    DcOn = int16(1);
    Enable     = int16(0);
    InverterOn = int16(0);
    Ready = int16(0);
    if(bInverterOn == 1||bQuitInverterOn == 0)
        DcOn = int16(0);
    end
end
